simulink model "thrust_weight_mass_IntegrationTest"  (R2014a)
settings: Solver=ode3  StartTime=0.0  StopTime=10.0  FixedStep=0.01  RelTol=1e-3
libraries: rocket_dynamic_data_library x3
settings Model: Creator=scorpii  LastModifiedBy=scorpii

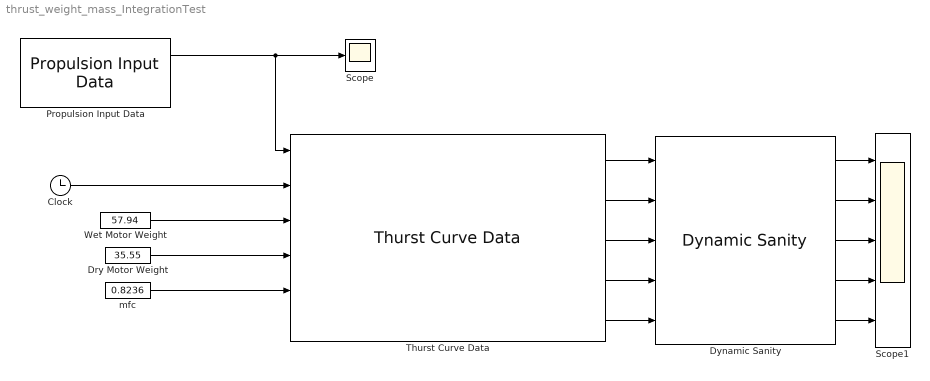
== system thrust_weight_mass_IntegrationTest ==
  Clock : Clock
  Dry Motor Weight : Constant  Value=35.55
  Dynamic Sanity : rocket_dynamic_data_library/Dynamic Sanity
  Propulsion Input Data : rocket_dynamic_data_library/Propulsion Input Data
  Scope : Scope
  Scope1 : Scope  NumInputPorts=5
      settings: YMin=-5~-5~-5~-5~-5  YMax=5~5~5~5~5
  Thurst Curve Data : rocket_dynamic_data_library/Thurst Curve Data
  Wet Motor Weight : Constant  Value=57.94
  mfc : Constant  Value=0.8236
  wires:
  Propulsion Input Data/1 -> Thurst Curve Data/1, Scope/1
  Clock/1 -> Thurst Curve Data/2
  Wet Motor Weight/1 -> Thurst Curve Data/3
  Dry Motor Weight/1 -> Thurst Curve Data/4
  mfc/1 -> Thurst Curve Data/5
  Thurst Curve Data/4 -> Dynamic Sanity/4
  Thurst Curve Data/1 -> Dynamic Sanity/1
  Thurst Curve Data/2 -> Dynamic Sanity/2
  Thurst Curve Data/3 -> Dynamic Sanity/3
  Thurst Curve Data/5 -> Dynamic Sanity/5
  Dynamic Sanity/5 -> Scope1/5
  Dynamic Sanity/1 -> Scope1/1
  Dynamic Sanity/2 -> Scope1/2
  Dynamic Sanity/4 -> Scope1/4
  Dynamic Sanity/3 -> Scope1/3
